simulink model "AW_test"  (R2015a)
settings: Solver=ode5  StartTime=0.0  StopTime=14  FixedStep=1e-4  RelTol=1e-3
values from neighbouring files (symbols this model uses):
  Ak = [815.666686466 -247.565739392 216455.990143 -40009.9793013 101833.013371 56966.4369443 -260.344441883 79.637972257 -70891.4834769 12846.1132956 -26185.98219 -17361.2721412 ... (36 elements, 6x6)]    [controller.mat]    (also in main_matlab_step1.m = rlqg.A)
  Ap = Ap(1:nn,1:nn)    [main_matlab_step1.m]    (also in plant.mat = [-0.773996386153 -96.4009703983 0 0 0 0 96.979553948 -1.6354)
  Bk = [-8.44020481469 2.14766413524 104.526982436 -93.1116400352 -68.3572551974 -11.8211224455]    [controller.mat]    (also in main_matlab_step1.m = rlqg.B)
  Bp = [-0.230745598618  -0.153904745996; 0.0612777559553  0.0606173681668; -25.0923163191  13.5416143638; 4.01556833701  -3.21559278869; -4.90371370695  20.5766878764; -5.44248661254  6.08611624326]    [plant.mat]
  Ck = [-6676.24518167  2388.66763685  162.329744068  -97.9536908458  -117.882548171  -121.1765543; 3434.83172263  -735.119667317  -67.5589205763  -7.32978906487  3.89518348807  52.6776382701]    [controller.mat]    (also in main_matlab_step1.m = rlqg.C)
  Cp = [-23.1554338545 9.56281796835 0.435674513054 -0.46619419818 -0.57533927079 -0.316369760482]    [plant.mat]
  Dk = [0 0]    [controller.mat]    (also in main_matlab_step1.m = rlqg.D)
  GAMA1 = [34.2579036952 -91.0423587876 0.025232839529 -0.0297347312876 0.00170993675498 -0.00975389455603 -0.0549933328975 -0.00162348051831 -0.000335321875448 4.62207436585e-05 -0.000828431634707 0.000271039057349 ... (144 elements, 12x12)]    [GAMA.mat]    (also in main_matlab_step3.m = GAMA(1:naw,1:naw); main_matlab_step3_test_for_delta.m = GAMA(1:naw,1:naw))
  GAMA2 = [-0.00119293833118 -0.000139352620147 0.000569164611738 -0.000680627504273 0.00211828949731 -0.00715334037597 -0.0351925855709 0.0168784094405 0.0214965617052 -0.0297469899893 0.0066102642616 -0.014985912494 ... (24 elements, 12x2)]    [GAMA.mat]    (also in main_matlab_step3.m = GAMA(1:naw,naw+1:end); main_matlab_step3_test_for_delta.m = GAMA(1:naw,naw+1:end))
  GAMA3 = [-2147.23436996 545.906876813 26602.1142963 -23617.9622211 -17413.9759172 -2975.51682709 0.00307933999877 -1.60845552356 81.2017993666 -20.7356427414 -1006.14734875 893.040945504 ... (96 elements, 8x12)]    [GAMA.mat]    (also in main_matlab_step3.m = GAMA(naw+1:end,1:naw); main_matlab_step3_test_for_delta.m = GAMA(naw+1:end,1:naw))
  GAMA4 = [0.00647719712126 -0.00238131629612 -0.000161503217854 0.000103315681118 0.00012320696114 0.000120218775716 -0.0663722306357 -0.00241762651299 -0.00325914135833 0.000649794705052 6.27880275548e-05 1.11393170952e-05 ... (16 elements, 8x2)]    [GAMA.mat]    (also in main_matlab_step3.m = GAMA(naw+1:end,naw+1:end); main_matlab_step3_test_for_delta.m = GAMA(naw+1:end,naw+1:end))
  Hp = [0.258916103899 0.10195659276 -1.80129126805 -4.56185147008 25.0926976513 -19.7319673467]    [plant.mat]
  nc = nk    [main_matlab_step1.m]    (also in main_matlab_step3.m = nn; main_matlab_step3_test_for_delta.m = nn)
  nu = numel(Bpu)/np    [main_matlab_step1.m]    (also in main_matlab_step3.m = 2; main_matlab_step3_test_for_delta.m = 2)
libraries: simulink x1
settings Model: Creator=p4wp4w  LastModifiedBy=p4wp4w

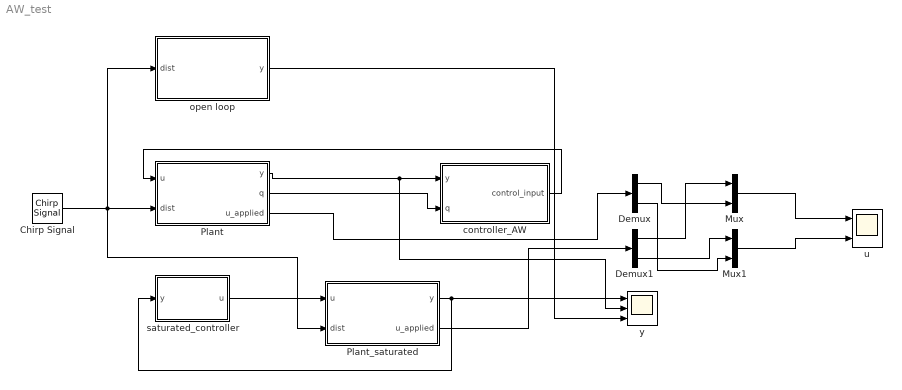
== system AW_test ==
  Chirp Signal : simulink/Sources/Chirp Signal  f1=0.1  T=14  f2=140
  Demux : Demux  Outputs=2
  Demux1 : Demux  Outputs=2
  Mux : Mux  Inputs=2
  Mux1 : Mux  Inputs=2
  Plant : Subsystem
  Plant_saturated : Subsystem
  controller_AW : Subsystem
  open loop : Subsystem
  "saturated_controller " : Subsystem
  u : Scope  NumInputPorts=2
      settings: YMin=-5~-5  YMax=5~5
  y : Scope  NumInputPorts=3
      settings: YMin=-5~-5~-5  YMax=5~5~5
  wires:
  Plant/1(y) -> y/2, controller_AW/1(y)
  Plant/2(q) -> controller_AW/2(q)
  controller_AW/1("control_input ") -> Plant/1(u)
  Chirp Signal/1 -> Plant_saturated/2(dist), open loop/1(dist), Plant/2(dist)
  "saturated_controller "/1(u) -> Plant_saturated/1(u)
  Plant_saturated/1(y) -> "saturated_controller "/1(y), y/1
  Demux1/1 -> Mux/1
  Demux/1 -> Mux/2
  Demux1/2 -> Mux1/1
  Demux/2 -> Mux1/2
  Mux/1 -> u/1
  Mux1/1 -> u/2
  Plant_saturated/2(u_applied) -> Demux1/1
  Plant/3(u_applied) -> Demux/1
  open loop/1(y) -> y/3

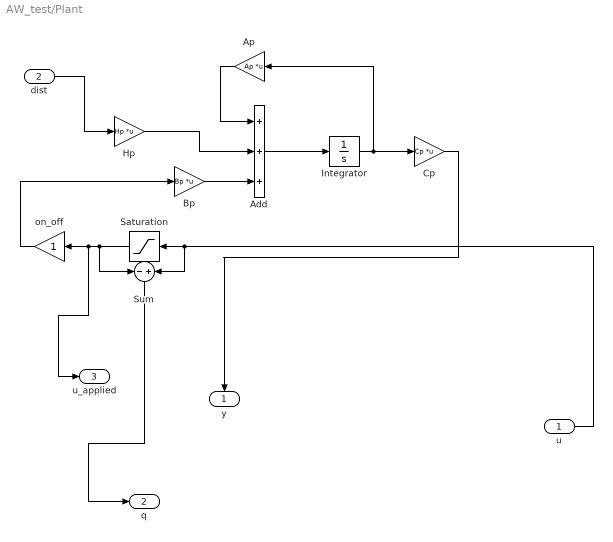
== system AW_test/Plant ==
  u : Inport
  dist : Inport  Port=2
  Add : Sum  Inputs=+++
  Ap : Gain  Gain=Ap  Multiplication=Matrix(K*u)
  Bp : Gain  Gain=Bp  Multiplication=Matrix(K*u)
  Cp : Gain  Gain=Cp  Multiplication=Matrix(K*u)
  Hp : Gain  Gain=Hp  Multiplication=Matrix(K*u)
  Integrator : Integrator
  Saturation : Saturate  UpperLimit=2  LowerLimit=-2
  Sum : Sum  Inputs=-|+
  on_off : Gain
  y : Outport
  q : Outport  Port=2
  u_applied : Outport  Port=3
  wires:
  Add/1 -> Integrator/1
  Cp/1 -> y/1
  Hp/1 -> Add/2
  on_off/1 -> Bp/1
  Integrator/1 -> Cp/1, Ap/1
  Saturation/1 -> Sum/1, u_applied/1, on_off/1
  Ap/1 -> Add/1
  u/1 -> Sum/2, Saturation/1
  Bp/1 -> Add/3
  Sum/1 -> q/1
  dist/1 -> Hp/1

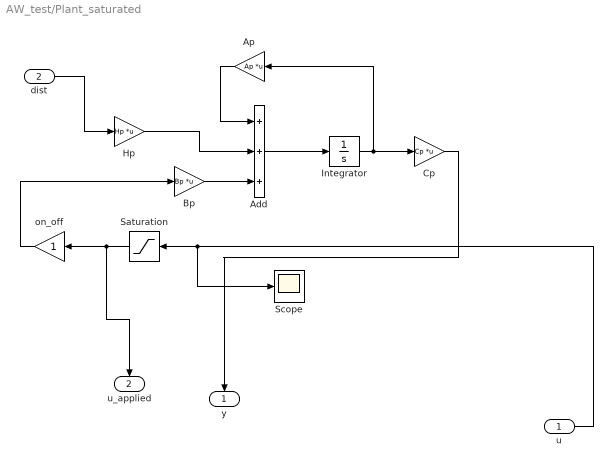
== system AW_test/Plant_saturated ==
  u : Inport
  dist : Inport  Port=2
  Add : Sum  Inputs=+++
  Ap : Gain  Gain=Ap  Multiplication=Matrix(K*u)
  Bp : Gain  Gain=Bp  Multiplication=Matrix(K*u)
  Cp : Gain  Gain=Cp  Multiplication=Matrix(K*u)
  Hp : Gain  Gain=Hp  Multiplication=Matrix(K*u)
  Integrator : Integrator
  Saturation : Saturate  UpperLimit=2  LowerLimit=-2
  Scope : Scope
      settings: YMin=-10  YMax=10  SaveName=ScopeData2
  on_off : Gain
  y : Outport
  u_applied : Outport  Port=2
  wires:
  dist/1 -> Hp/1
  Bp/1 -> Add/3
  u/1 -> Scope/1, Saturation/1
  Ap/1 -> Add/1
  Saturation/1 -> u_applied/1, on_off/1
  Integrator/1 -> Ap/1, Cp/1
  on_off/1 -> Bp/1
  Hp/1 -> Add/2
  Cp/1 -> y/1
  Add/1 -> Integrator/1

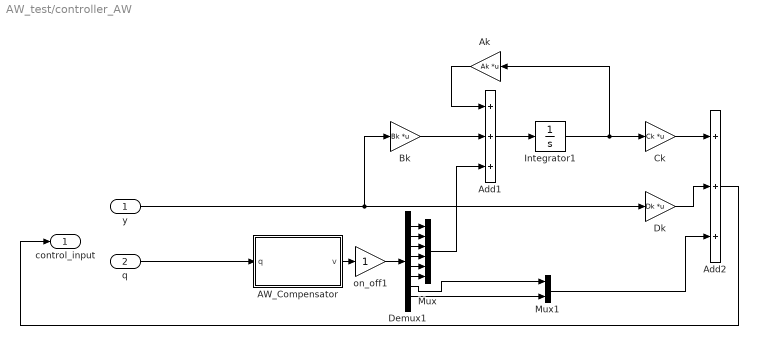
== system AW_test/controller_AW ==
  y : Inport
  q : Inport  Port=2
  AW_Compensator : Subsystem
  Add1 : Sum  Inputs=+++
  Add2 : Sum  Inputs=+++
  Ak : Gain  Gain=Ak  Multiplication=Matrix(K*u)
  Bk : Gain  Gain=Bk  Multiplication=Matrix(K*u)
  Ck : Gain  Gain=Ck  Multiplication=Matrix(K*u)
  Demux1 : Demux  Outputs=nc+nu
  Dk : Gain  Gain=Dk  Multiplication=Matrix(K*u)
  Integrator1 : Integrator
  Mux : Mux  Inputs=nc
  Mux1 : Mux  Inputs=nu
  on_off1 : Gain
  "control_input " : Outport
  wires:
  Demux1/1 -> Mux/1
  Demux1/2 -> Mux/2
  Ck/1 -> Add2/1
  Demux1/8 -> Mux1/2
  Add1/1 -> Integrator1/1
  Ak/1 -> Add1/1
  AW_Compensator/1(v) -> on_off1/1
  Bk/1 -> Add1/2
  Demux1/3 -> Mux/3
  Integrator1/1 -> Ck/1, Ak/1
  Dk/1 -> Add2/2
  Demux1/7 -> Mux1/1
  Demux1/4 -> Mux/4
  Demux1/6 -> Mux/6
  Demux1/5 -> Mux/5
  on_off1/1 -> Demux1/1
  Mux1/1 -> Add2/3
  Mux/1 -> Add1/3
  y/1 -> Bk/1, Dk/1
  q/1 -> AW_Compensator/1(q)
  Add2/1 -> "control_input "/1

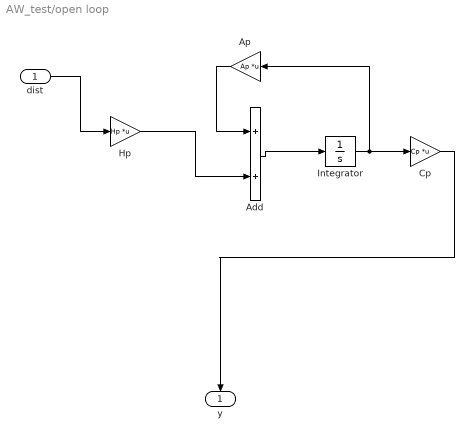
== system AW_test/open loop ==
  dist : Inport
  Add : Sum
  Ap : Gain  Gain=Ap  Multiplication=Matrix(K*u)
  Cp : Gain  Gain=Cp  Multiplication=Matrix(K*u)
  Hp : Gain  Gain=Hp  Multiplication=Matrix(K*u)
  Integrator : Integrator
  y : Outport
  wires:
  dist/1 -> Hp/1
  Ap/1 -> Add/1
  Integrator/1 -> Ap/1, Cp/1
  Hp/1 -> Add/2
  Cp/1 -> y/1
  Add/1 -> Integrator/1

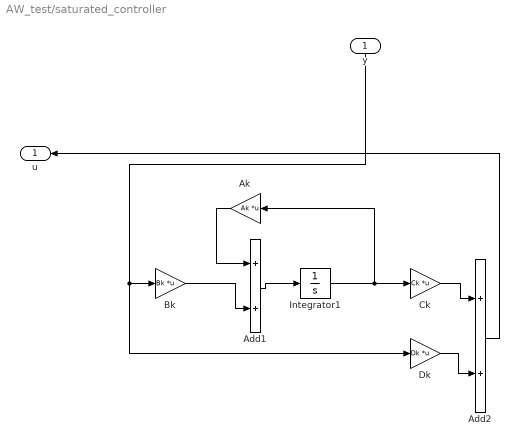
== system AW_test/saturated_controller  ==
  y : Inport
  Add1 : Sum
  Add2 : Sum
  Ak : Gain  Gain=Ak  Multiplication=Matrix(K*u)
  Bk : Gain  Gain=Bk  Multiplication=Matrix(K*u)
  Ck : Gain  Gain=Ck  Multiplication=Matrix(K*u)
  Dk : Gain  Gain=Dk  Multiplication=Matrix(K*u)
  Integrator1 : Integrator
  u : Outport
  wires:
  Bk/1 -> Add1/2
  Add1/1 -> Integrator1/1
  Ck/1 -> Add2/1
  Dk/1 -> Add2/2
  Integrator1/1 -> Ck/1, Ak/1
  Add2/1 -> u/1
  Ak/1 -> Add1/1
  y/1 -> Bk/1, Dk/1

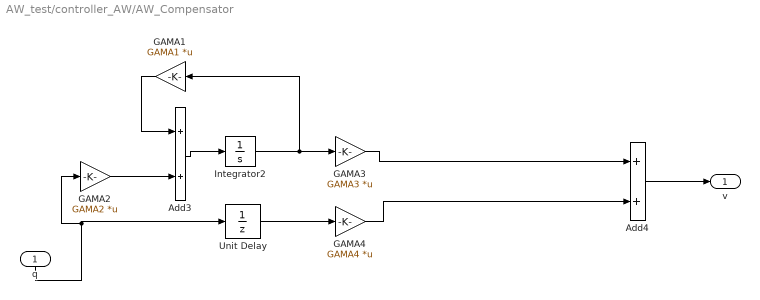
== system AW_test/controller_AW/AW_Compensator ==
  q : Inport
  Add3 : Sum
  Add4 : Sum
  GAMA1 : Gain  Gain=GAMA1  Multiplication=Matrix(K*u)
  GAMA2 : Gain  Gain=GAMA2  Multiplication=Matrix(K*u)
  GAMA3 : Gain  Gain=GAMA3  Multiplication=Matrix(K*u)
  GAMA4 : Gain  Gain=GAMA4  Multiplication=Matrix(K*u)
  Integrator2 : Integrator
  Unit Delay : UnitDelay  SampleTime=-1
  v : Outport
  wires:
  Add3/1 -> Integrator2/1
  GAMA3/1 -> Add4/1
  GAMA1/1 -> Add3/1
  Integrator2/1 -> GAMA3/1, GAMA1/1
  GAMA2/1 -> Add3/2
  GAMA4/1 -> Add4/2
  Add4/1 -> v/1
  q/1 -> Unit Delay/1, GAMA2/1
  Unit Delay/1 -> GAMA4/1
